simulink model "sysgenPolyphaseChannelizer"  (Simulink 7.7)
settings: Solver=VariableStepDiscrete  StartTime=0.0  StopTime=200000.0  RelTol=1e-3
values from neighbouring files (symbols this model uses):
  Fs = 1 ./ block_data.params.XIncr    [sdspfscope2_r13.m]
undefined symbols (not defined in the file or in its folder): sided, Two, xlfda_numerator, xlipgetpartsetting
libraries: xbsIndex_r4 x37, dspsigops x6, dspsrcs4 x3, dspsnks4 x2, simulink x1, xbsCopyrightNotice_r4 x1
settings Model: Creator=andrewd  LastModifiedBy=arvinds
settings OptimizationCC: InitFltsAndDblsToZero=on
settings DebuggingCC: SaveWithParameterizedLinksMsg=none  SignalResolutionControl=TryResolveAllWithWarning  StrictBusMsg=Warning
settings GRTTargetCC: TargetFcnLib=ansi_tfl_tmw.mat

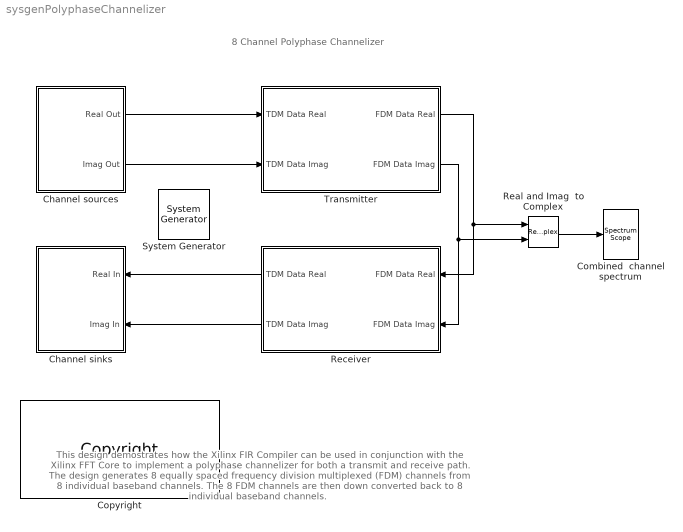
== system sysgenPolyphaseChannelizer ==
  note: 8 Channel Polyphase Channelizer
  note: This design demostrates how the Xilinx FIR Compiler can be used
      | in conjunction with the Xilinx FFT Core to implement a polyphase
      | channelizer for both a transmit and receive path.
      |
      | The design generates 8 equally spaced frequency division multiplexed
      | (FDM) channels from 8 individual baseband channels. The 8 FDM
      | channels are then down converted back to 8 individual baseband
      | channels.
  " System Generator" : xbsIndex_r4/ System Generator  Tag=genX  SystemSampleTime=-1  xilinxfamily=virtex6  part=xc6vlx240t  speed=-1  package=ff1156  synthesis_tool=XST  clock_wrapper=Clock Enables  directory=./timing  proj_type=Project Navigator  Synth_file=XST Defaults  Impl_file=ISE Defaults  testbench=off  simulink_period=1  sysclk_period=1e9/(length(xlfda_numerator([bdroot,'/Transmitter/FDATool']))*200e3)  dcm_input_clock_period=100  incr_netlist=off  trim_vbits=Everywhere in SubSystem  dbl_ovrd=According to Block Masks  core_generation=According to Block Masks  run_coregen=off  deprecated_control=off  eval_field=0  block_type=sysgen
      settings: block_version=10.1.2
  Channel sinks : Subsystem
  Channel sources : Subsystem
  Combined  channel spectrum : dspsnks4/Spectrum Scope  SystemSampleTime=-1  ScopeProperties=on  Domain=Frequency  HorizSpan=1  UseBuffer=on  BufferSize=512  Overlap=0  TreatMby1Signals=M channels  inpFftLenInherit=on  FFTlength=512  numAvg=2  DisplayProperties=off  AxisGrid=on  Memory=off  FrameNumber=on  AxisLegend=off  AxisZoom=off  OpenScopeAtSimStart=on  OpenScopeImmediately=off  FigPos=[-726 581 381 243]  AxisProperties=off  XUnits=Hertz  XRange=Two-sided ((-Fs/2...Fs/2])  XDisplay=0  InheritXIncr=on  XIncr=1.0  XLabel=Samples  XLimit=User-defined  YUnits=dBm/Hertz  XMax=0.005618  XMin=-0.005618  YLabel=Magnitude-squared, dB  LineProperties=off  wintypeSpecScope=Hann  RsSpecScope=50  betaSpecScope=5  winsampSpecScope=Periodic  XAxisParamsVer=6.8  isFrameUpgraded=on
      settings: YMin=-112.1379  YMax=9.2197
  Copyright : xbsCopyrightNotice_r4/Copyright  copyrighttext="Copyright (c) 2011  by  Xilinx, Inc. All rights reserved.<br><br>This file contains proprietary, confidential information of Xilinx, Inc., is distributed under license from Xilinx, Inc., and may be used, copied and/or disclosed only pursuant to the terms of a valid license agreement with Xilinx, Inc. Xilinx hereby grants you a license to use this file solely for design, simulation, implementation and creation of design files limited to Xilinx devices or technologies. Use with non-Xilinx devices or technologies is expressly prohibited and immediately terminates your license unless covered by a separate agreement.<br><br>Xilinx is providing this design, code, or information \"as-is\" solely for use in developing programs and solutions for Xilinx devices, with no obligation on the part of Xilinx to provide support. By providing this design, code, or information as one possible implementation of this feature, application or standard, Xilinx is making no representation that this implementation is free from any claims of infringement. You are responsible for obtaining any rights you may require for your implementation. Xilinx expressly disclaims any warranty whatsoever with respect to the adequacy of the implementation, including but not limited to any warranties or representations that this implementation is free from claims of infringement, implied warranties of merchantability or fitness for a particular purpose.<br><br>Xilinx products are not intended for use in life support appliances, devices, or systems. Use in such applications is expressly prohibited.<br><br>Any modifications that are made to the Source Code are done at the user's sole risk and will be unsupported.<br><br>This copyright and support notice must be retained as part of this text at all times. (c) Copyright 1995-2011 Xilinx, Inc. All rights reserved."  block_type=copyright
      settings: block_version=10.1.2
      settings: infoedit=|
      | Copyright(C) 2008 by  Xilinx, Inc. All rights reserved.<br>
      | <br>
      | This file contains proprietary, confidential information of Xilinx, Inc., is distributed under license
      | from Xilinx, Inc., and may be used, copied and/or disclosed only pursuant to the terms of a valid license
      | agreement with Xilinx, Inc. Xilinx hereby grants you a license to use this file solely for design,
      | simulation, implementation and creation of design files limited to Xilinx devices or technologies. Use
      | with non-Xilinx devices or technologies is expressly prohibited and immediately terminates your license
      | unless covered by a separate agreement.<br>
      | <br>
      | Xilinx is providing this design, code, or information "as-is" solely for use in developing programs and
      | solutions for Xilinx devices, with no obligation on the part of Xilinx to provide support. By providing
      | this design, code, or information as one possible implementation of this feature, application or standard,
      | Xilinx is making no representation that this implementation is free from any claims of infringement. You
      | are responsible for obtaining any rights you may require for your implementation. Xilinx expressly disclaims
      | any warranty whatsoever with respect to the adequacy of the implementation, including but not limited to any
      | warranties or representations that this implementation is free from claims of infringement, implied warranties
      | of merchantability or fitness for a particular purpose.<br>
      | <br>
      | Xilinx products are not intended for use in life support appliances, devices, or systems. Use in such
      | applications is expressly prohibited.<br>
      | <br>
      | Any modifications that are made to the Source Code are done at the user's sole risk and will be unsupported.<br>
      | <br>
      | This copyright and support notice must be retained as part of this text at all times.
      | (c) Copyright 1995-2008 Xilinx, Inc. All rights reserved.
  Real and Imag  to Complex : RealImagToComplex
  Receiver : Subsystem
  Transmitter : Subsystem
  wires:
  Channel sources/1(Real Out) -> Transmitter/1(TDM Data Real)
  Channel sources/2(Imag Out) -> Transmitter/2(TDM Data Imag)
  Real and Imag  to Complex/1 -> Combined  channel spectrum/1
  Transmitter/1(FDM Data Real) -> Receiver/1(FDM Data Real), Real and Imag  to Complex/1
  Transmitter/2(FDM Data Imag) -> Receiver/2(FDM Data Imag), Real and Imag  to Complex/2
  Receiver/1(TDM Data Real) -> Channel sinks/1(Real In)
  Receiver/2(TDM Data Imag) -> Channel sinks/2(Imag In)

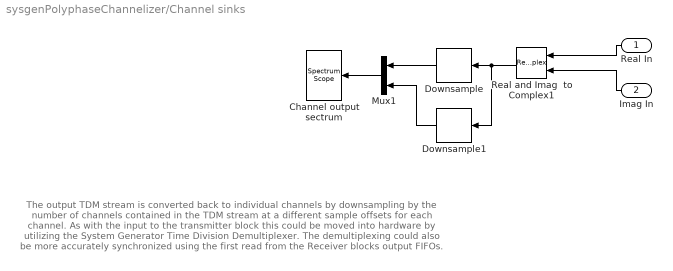
== system sysgenPolyphaseChannelizer/Channel sinks ==
  note: The output TDM stream is converted back to individual channels
      | by downsampling by the number of channels contained in the TDM
      | stream at a different sample offsets for each channel. As with the
      | input to the transmitter block this could be moved into hardware
      | by utilizing the System Generator Time Division Demultiplexer. The
      | demultiplexing could also be more accurately synchronized using
      | the first read from the Receiver blocks output FIFOs.
  Real In : Inport
  Imag In : Inport  Port=2
  Channel output sectrum : dspsnks4/Spectrum Scope  SystemSampleTime=-1  ScopeProperties=on  Domain=Frequency  HorizSpan=1  UseBuffer=on  BufferSize=256  Overlap=0  TreatMby1Signals=M channels  inpFftLenInherit=off  FFTlength=128  numAvg=2  DisplayProperties=off  AxisGrid=on  Memory=off  FrameNumber=on  AxisLegend=on  AxisZoom=off  OpenScopeAtSimStart=on  OpenScopeImmediately=off  FigPos=[-742 232 386 238]  AxisProperties=off  XUnits=Hertz  XRange=Two-sided ((-Fs/2...Fs/2])  XDisplay=0  InheritXIncr=on  XIncr=1.0  XLabel=Samples  XLimit=Auto  YUnits=dBm/Hertz  XMax=0.00070225  XMin=-0.00070225  YLabel=Magnitude-squared, dB  LineProperties=off  LineColors=[1 0 0]  wintypeSpecScope=Hann  RsSpecScope=50  betaSpecScope=5  winsampSpecScope=Periodic  XAxisParamsVer=6.9  isFrameUpgraded=on
      settings: YMin=-79.5628  YMax=47.0211
  Downsample : dspsigops/Downsample  N=8  phase=4  InputProcessing=Inherited (this choice will be removed - see release notes)  RateOptions=Enforce single-rate processing  smode=Allow multirate  fmode=Maintain input frame size  ic=0
  Downsample1 : dspsigops/Downsample  N=8  phase=0  InputProcessing=Inherited (this choice will be removed - see release notes)  RateOptions=Enforce single-rate processing  smode=Allow multirate  fmode=Maintain input frame size  ic=0
  Mux1 : Mux  Inputs=2
  Real and Imag  to Complex1 : RealImagToComplex
  wires:
  Real and Imag  to Complex1/1 -> Downsample/1, Downsample1/1
  Mux1/1 -> Channel output sectrum/1
  Downsample/1 -> Mux1/1
  Downsample1/1 -> Mux1/2
  Real In/1 -> Real and Imag  to Complex1/1
  Imag In/1 -> Real and Imag  to Complex1/2

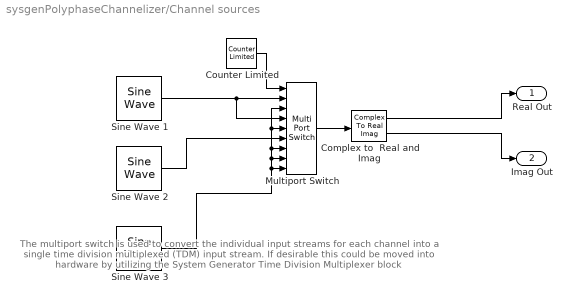
== system sysgenPolyphaseChannelizer/Channel sources ==
  note: The multiport switch is used to convert the individual input streams
      | for each channel into a single time division multiplexed (TDM)
      | input stream. If desirable this could be moved into hardware by
      | utilizing the System Generator Time Division Multiplexer block
  Complex to  Real and Imag : ComplexToRealImag
  Counter Limited : simulink/Sources/Counter Limited  SystemSampleTime=-1  uplimit=7  tsamp=length(xlfda_numerator([bdroot,'/Transmitter/FDATool']))/8
  Multiport Switch : MultiPortSwitch  DataPortOrder=Zero-based contiguous  Inputs=8  zeroidx=on  InputSameDT=on
  Sine Wave 1 : dspsrcs4/Sine Wave  Amplitude=1  Frequency=11.23456e3/(200e3*length(xlfda_numerator([bdroot,'/Transmitter/FDATool'])))  Phase=0  SampleMode=Discrete  OutComplex=Complex  CompMethod=Trigonometric fcn  TableSize=Speed  SampleTime=length(xlfda_numerator([bdroot,'/Transmitter/FDATool']))  SamplesPerFrame=1  ResetState=Restart at time zero  dataType=double  wordLen=16  udDataType=sfix(16)  fracBitsMode=Best precision  numFracBits=15  OutDataTypeStr=double  LastOutDataTypeStr=double
  Sine Wave 2 : dspsrcs4/Sine Wave  Amplitude=0.5  Frequency=50.234567e3/(200e3*length(xlfda_numerator([bdroot,'/Transmitter/FDATool'])))  Phase=0  SampleMode=Discrete  OutComplex=Complex  CompMethod=Trigonometric fcn  TableSize=Speed  SampleTime=length(xlfda_numerator([bdroot,'/Transmitter/FDATool']))  SamplesPerFrame=1  ResetState=Restart at time zero  dataType=double  wordLen=16  udDataType=sfix(16)  fracBitsMode=Best precision  numFracBits=15  OutDataTypeStr=double  LastOutDataTypeStr=double
  Sine Wave 3 : dspsrcs4/Sine Wave  Amplitude=0  Frequency=0  Phase=0  SampleMode=Discrete  OutComplex=Complex  CompMethod=Trigonometric fcn  TableSize=Speed  SampleTime=length(xlfda_numerator([bdroot,'/Transmitter/FDATool']))  SamplesPerFrame=1  ResetState=Restart at time zero  dataType=double  wordLen=16  udDataType=sfix(16)  fracBitsMode=Best precision  numFracBits=15  OutDataTypeStr=double  LastOutDataTypeStr=double
  Real Out : Outport
  Imag Out : Outport  Port=2
  wires:
  Multiport Switch/1 -> Complex to  Real and Imag/1
  Sine Wave 1/1 -> Multiport Switch/2, Multiport Switch/4
  Counter Limited/1 -> Multiport Switch/1
  Sine Wave 2/1 -> Multiport Switch/6
  Sine Wave 3/1 -> Multiport Switch/8, Multiport Switch/7, Multiport Switch/5, Multiport Switch/3, Multiport Switch/9
  Complex to  Real and Imag/1 -> Real Out/1
  Complex to  Real and Imag/2 -> Imag Out/1

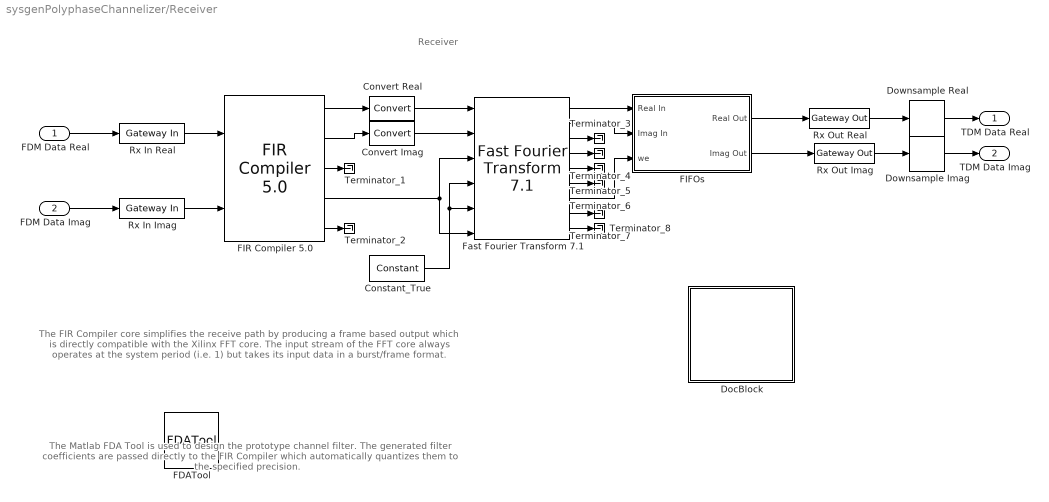
== system sysgenPolyphaseChannelizer/Receiver ==
  note: The FIR Compiler core simplifies the receive path by producing a frame
      | based output which is directly compatible with the Xilinx FFT core.
      | The input stream of the FFT core always operates at the system
      | period (i.e. 1) but takes its input data in a burst/frame format.
  note: Receiver
  note: The Matlab FDA Tool is used to design the prototype
      | channel filter. The generated filter coefficients are
      | passed directly to the FIR Compiler which
      | automatically quantizes them to the specified
      | precision.
  FDM Data Real : Inport
  FDM Data Imag : Inport  Port=2
  Constant_True : xbsIndex_r4/Constant  const=1  gui_display_data_type=Fixed-point  arith_type=Boolean  n_bits=16  bin_pt=14  preci_type=Single  exp_width=8  frac_width=24  explicit_period=on  period=1  equ=P=C  opselect=C  inp2=PCIN>>17  opr=+  inp1=P  carry=CIN  dbl_ovrd=off  block_type=constant
      settings: block_version=10.1.2
  Convert Imag : xbsIndex_r4/Convert  gui_display_data_type=Fixed-point  arith_type="Signed  (2's comp)"  n_bits=17  bin_pt=16  float_type=Single  exp_bits=8  fraction_bits=24  quantization=Truncate  overflow=Wrap  en=off  latency=0  dbl_ovrd=off  pipeline=off  block_type=convert
      settings: block_version=10.1.2
  Convert Real : xbsIndex_r4/Convert  gui_display_data_type=Fixed-point  arith_type="Signed  (2's comp)"  n_bits=17  bin_pt=16  float_type=Single  exp_bits=8  fraction_bits=24  quantization=Truncate  overflow=Wrap  en=off  latency=0  dbl_ovrd=off  pipeline=off  block_type=convert
      settings: block_version=10.1.2
  DocBlock : Subsystem  AncestorBlock=simulink/Model-Wide Utilities/DocBlock  mask(DocBlock){ECoderFlag=, DocumentType=RTF}
      mask prompts: ECoderFlag "RTW Embedded Coder Flag"; DocumentType "Document Type"
      mask help: Use this block to save long descriptive text with the model. Double-clicking the block will open an editor.
      settings: DeleteFcn=docblock('close_document',gcb);  PreSaveFcn=docblock('save_document',gcb);  OpenFcn=docblock('edit_document',gcb);
      mask StyleString: edit,popup(Text|RTF|HTML)
      mask Display:
      | plot([.8 0 0 1 1 .8 .8 1],[1 1 0 0 .8 1 .8 .8]);
      | text(.5,.6,'Double click\n for more information','horizontalalignment','center');
  Downsample Imag : dspsigops/Downsample  N=length(xlfda_numerator('FDATool'))/8  phase=0  InputProcessing=Inherited (this choice will be removed - see release notes)  RateOptions=Enforce single-rate processing  smode=Allow multirate  fmode=Maintain input frame size  ic=0
  Downsample Real : dspsigops/Downsample  N=length(xlfda_numerator('FDATool'))/8  phase=0  InputProcessing=Inherited (this choice will be removed - see release notes)  RateOptions=Enforce single-rate processing  smode=Allow multirate  fmode=Maintain input frame size  ic=0
  FDATool : xbsIndex_r4/FDATool  block_type=fdatool
      settings: infoedit=FDATool  block_version=10.1.2
  FIFOs : Subsystem
  "FIR Compiler 5.0 " : xbsIndex_r4/FIR Compiler 5.0   coefficientvector=8.*xlfda_numerator('FDATool')  coefficient_sets=1  filter_type=Polyphase_Filter_Bank_Receiver  rate_change_type=Integer  interpolation_rate=1  decimation_rate=1  zero_pack_factor=1  number_channels=8  ratespecification=Maximum_Possible  sampleperiod=1  hardwareoversamplingrate=1  filter_architecture=Systolic_Multiply_Accumulate  coefficient_reload=off  coefficient_structure=Non_Symmetric  coefficient_sign=Signed  quantization=Quantize_Only  coefficient_width=25  bestprecision=off  coefficient_fractional_bits=24  number_paths=2  output_rounding_mode=Convergent_Rounding_to_Even  output_width=19  allow_rounding_approximation=off  optimization_goal=Area  has_sclr=off  has_data_valid=off  has_nd=off  has_ce=off  usechan_in_adv=off  chan_in_adv=0  data_buffer_type=Automatic  coefficient_buffer_type=Automatic  input_buffer_type=Automatic  output_buffer_type=Automatic  preference_for_other_storage=Automatic  multi_column_support=Automatic  columnconfig='32,32,25'  inter_column_pipe_length=4  passband_min=0.0  passband_max=0.5  stopband_min=0.5  stopband_max=1.0  filter_selection=1  gui_behaviour=Sysgen  registered_output=true  data_sign=Signed  data_width=16  data_fractional_bits=0  wrapper_available=true  ip_wrap_arbitrary_binary_point=true  ip_name=FIR Compiler  ip_version=5.0  dsptool_ready=true  ipcore_usecache=true  ipcore_useipmodelcache=true  ipcore_xco_need_fpga_part=true  port_translation_map={ 'ce' => 'en', 'sclr' => 'rst' }  run_core_at_system_period=true  ipcore_fpga_part=xlipgetpartsetting(gcb, {'virtex4', 'xc4vsx35', '-10', 'ff668'})  structural_sim=false  block_type=fir_compiler_v5_0
      settings: block_version=11.1.2
  "Fast Fourier Transform 7.1 " : xbsIndex_r4/Fast Fourier Transform 7.1   transform_length=8  implementation_options=radix_2_lite_burst_io  target_clock_frequency=250  target_data_throughput=50  run_time_configurable_transform_length=off  phase_factor_width=17  scaling_options=unscaled  rounding_modes=convergent_rounding  output_ordering=natural_order  cyclic_prefix_insertion=off  ce=off  sclr=off  ovflo=off  input_data_offset=three_cycle_offset  memory_options_data=distributed_ram  memory_options_phase_factors=distributed_ram  number_of_stages_using_block_ram_for_data_and_phase_factors=0  memory_options_reorder=block_ram  memory_options_hybrid=off  complex_mult_type=use_mults_performance  butterfly_type=use_xtremedsp_slices  channels=1  input_ordering=natural_order  input_width=16  simulation_type=external_xfix  simulation_model=fftv71_CModel:fftv71_cmodel  ip_name=Fast Fourier Transform  ip_version=7.1  dsptool_ready=true  wrapper_available=true  port_translation_map={ 'ce' => 'en', 'sclr' => 'rst' }  ipcore_fpga_part=xlipgetpartsetting(gcb, {'virtex4', 'xc4vsx35', '-10', 'ff668'})  block_type=xfft_v7_1
      settings: block_version=12.1
  Rx In Imag : xbsIndex_r4/Gateway In  gui_display_data_type=Fixed-point  arith_type="Signed  (2's comp)"  n_bits=16  bin_pt=15  preci_type=Single  exp_width=8  frac_width=24  quantization="Round  (unbiased: +/- Inf)"  overflow=Saturate  period=length(xlfda_numerator('FDATool'))/8  dbl_ovrd=off  timing_constraint=None  locs_specified=off  LOCs={}  inherit_from_input=off  UseAsADC=off  ADCChannel='1'  hdl_port=on  block_type=gatewayin
      settings: infoedit="Gateway in block.  Converts inputs of type Simulink integer, double and fixed point to  Xilinx fixed point type.<P><P>Hardware notes:  In hardware these blocks become top level input ports."  block_version=10.1.2
  Rx In Real : xbsIndex_r4/Gateway In  gui_display_data_type=Fixed-point  arith_type="Signed  (2's comp)"  n_bits=16  bin_pt=15  preci_type=Single  exp_width=8  frac_width=24  quantization="Round  (unbiased: +/- Inf)"  overflow=Saturate  period=length(xlfda_numerator('FDATool'))/8  dbl_ovrd=off  timing_constraint=None  locs_specified=off  LOCs={}  inherit_from_input=off  UseAsADC=off  ADCChannel='1'  hdl_port=on  block_type=gatewayin
      settings: infoedit="Gateway in block.  Converts inputs of type Simulink integer, double and fixed point to  Xilinx fixed point type.<P><P>Hardware notes:  In hardware these blocks become top level input ports."  block_version=10.1.2
  Rx Out Imag : xbsIndex_r4/Gateway Out  inherit_from_input=off  hdl_port=on  timing_constraint=None  locs_specified=off  LOCs={}  UseAsDAC=off  DACChannel='1'  block_type=gatewayout
      settings: infoedit="Gateway out block.  Converts Xilinx fixed point inputs into ouputs of type Simulink integer, double, or fixed point.<P><P>Hardware notes:  In hardware these blocks become top level output ports or are discarded, depending on how they are configured."  block_version=10.1.2
  Rx Out Real : xbsIndex_r4/Gateway Out  inherit_from_input=off  hdl_port=on  timing_constraint=None  locs_specified=off  LOCs={}  UseAsDAC=off  DACChannel='1'  block_type=gatewayout
      settings: infoedit="Gateway out block.  Converts Xilinx fixed point inputs into ouputs of type Simulink integer, double, or fixed point.<P><P>Hardware notes:  In hardware these blocks become top level output ports or are discarded, depending on how they are configured."  block_version=10.1.2
  Terminator_{1..8} (8 alike) : Terminator
  TDM Data Real : Outport
  TDM Data Imag : Outport  Port=2
  wires:
  FDM Data Real/1 -> Rx In Real/1
  FDM Data Imag/1 -> Rx In Imag/1
  Rx In Real/1 -> "FIR Compiler 5.0 "/1
  Rx In Imag/1 -> "FIR Compiler 5.0 "/2
  "FIR Compiler 5.0 "/1 -> Convert Real/1
  "FIR Compiler 5.0 "/2 -> Convert Imag/1
  Constant_True/1 -> "Fast Fourier Transform 7.1 "/5, "Fast Fourier Transform 7.1 "/4
  Convert Real/1 -> "Fast Fourier Transform 7.1 "/1
  Convert Imag/1 -> "Fast Fourier Transform 7.1 "/2
  "FIR Compiler 5.0 "/4 -> "Fast Fourier Transform 7.1 "/6, "Fast Fourier Transform 7.1 "/3
  "Fast Fourier Transform 7.1 "/1 -> FIFOs/1(Real In)
  "Fast Fourier Transform 7.1 "/2 -> FIFOs/2(Imag In)
  "Fast Fourier Transform 7.1 "/7 -> FIFOs/3(we)
  FIFOs/1(Real Out) -> Rx Out Real/1
  FIFOs/2(Imag Out) -> Rx Out Imag/1
  Rx Out Real/1 -> Downsample Real/1
  Rx Out Imag/1 -> Downsample Imag/1
  "FIR Compiler 5.0 "/3 -> Terminator_1/1
  "FIR Compiler 5.0 "/5 -> Terminator_2/1
  "Fast Fourier Transform 7.1 "/3 -> Terminator_3/1
  "Fast Fourier Transform 7.1 "/4 -> Terminator_4/1
  "Fast Fourier Transform 7.1 "/5 -> Terminator_5/1
  "Fast Fourier Transform 7.1 "/6 -> Terminator_6/1
  "Fast Fourier Transform 7.1 "/8 -> Terminator_7/1
  "Fast Fourier Transform 7.1 "/9 -> Terminator_8/1
  Downsample Real/1 -> TDM Data Real/1
  Downsample Imag/1 -> TDM Data Imag/1

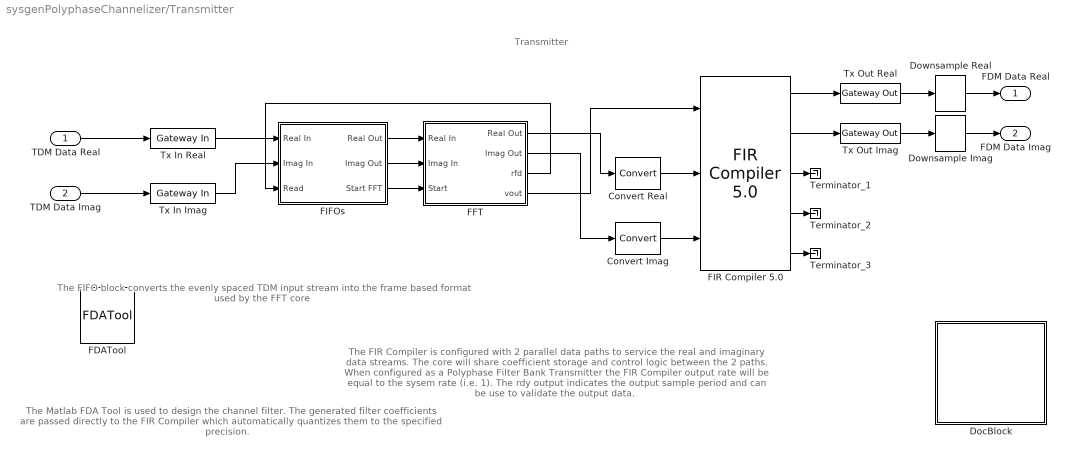
== system sysgenPolyphaseChannelizer/Transmitter ==
  note: The FIFO block converts the evenly spaced
      | TDM input stream into the frame based format
      | used by the FFT core
  note: The FIR Compiler is configured with 2 parallel data paths
      | to service the real and imaginary data streams. The core will
      | share coefficient storage and control logic between the 2 paths.
      | When configured as a Polyphase Filter Bank Transmitter the
      | FIR Compiler output rate will be equal to the sysem rate (i.e. 1).
      | The rdy output indicates the output sample period and can be
      | use to validate the output data.
  note: Transmitter
  note: The Matlab FDA Tool is used to design the
      | channel filter. The generated filter coefficients are
      | passed directly to the FIR Compiler which
      | automatically quantizes them to the specified
      | precision.
  TDM Data Real : Inport
  TDM Data Imag : Inport  Port=2
  Convert Imag : xbsIndex_r4/Convert  gui_display_data_type=Fixed-point  arith_type="Signed  (2's comp)"  n_bits=18  bin_pt=13  float_type=Single  exp_bits=8  fraction_bits=24  quantization="Round  (unbiased: Even Values)"  overflow=Wrap  en=off  latency=0  dbl_ovrd=off  pipeline=off  block_type=convert
      settings: block_version=10.1.2
  Convert Real : xbsIndex_r4/Convert  gui_display_data_type=Fixed-point  arith_type="Signed  (2's comp)"  n_bits=18  bin_pt=13  float_type=Single  exp_bits=8  fraction_bits=24  quantization="Round  (unbiased: Even Values)"  overflow=Wrap  en=off  latency=0  dbl_ovrd=off  pipeline=off  block_type=convert
      settings: block_version=10.1.2
  DocBlock : Subsystem  AncestorBlock=simulink/Model-Wide Utilities/DocBlock  mask(DocBlock){ECoderFlag=, DocumentType=RTF}
      mask prompts: ECoderFlag "RTW Embedded Coder Flag"; DocumentType "Document Type"
      mask help: Use this block to save long descriptive text with the model. Double-clicking the block will open an editor.
      settings: DeleteFcn=docblock('close_document',gcb);  PreSaveFcn=docblock('save_document',gcb);  OpenFcn=docblock('edit_document',gcb);
      mask StyleString: edit,popup(Text|RTF|HTML)
      mask Display:
      | plot([.8 0 0 1 1 .8 .8 1],[1 1 0 0 .8 1 .8 .8]);
      | text(.5,.6,'Double click\n for more information','horizontalalignment','center');
  Downsample Imag : dspsigops/Downsample  N=length(xlfda_numerator('FDATool'))/8  phase=0  InputProcessing=Inherited (this choice will be removed - see release notes)  RateOptions=Enforce single-rate processing  smode=Allow multirate  fmode=Maintain input frame size  ic=0
  Downsample Real : dspsigops/Downsample  N=length(xlfda_numerator('FDATool'))/8  phase=0  InputProcessing=Inherited (this choice will be removed - see release notes)  RateOptions=Enforce single-rate processing  smode=Allow multirate  fmode=Maintain input frame size  ic=0
  FDATool : xbsIndex_r4/FDATool  block_type=fdatool
      settings: infoedit=FDATool  block_version=10.1.2
  FFT : Subsystem
  FIFOs : Subsystem
  "FIR Compiler 5.0 " : xbsIndex_r4/FIR Compiler 5.0   coefficientvector=xlfda_numerator('FDATool')  coefficient_sets=1  filter_type=Polyphase_Filter_Bank_Transmitter  rate_change_type=Integer  interpolation_rate=1  decimation_rate=1  zero_pack_factor=1  number_channels=8  ratespecification=Sample_Period  sampleperiod=length(xlfda_numerator('FDATool'))/8  hardwareoversamplingrate=1  filter_architecture=Systolic_Multiply_Accumulate  coefficient_reload=off  coefficient_structure=Non_Symmetric  coefficient_sign=Signed  quantization=Quantize_Only  coefficient_width=25  bestprecision=off  coefficient_fractional_bits=27  number_paths=2  output_rounding_mode=Convergent_Rounding_to_Odd  output_width=19  allow_rounding_approximation=off  optimization_goal=Area  has_sclr=off  has_data_valid=off  has_nd=on  has_ce=off  usechan_in_adv=off  chan_in_adv=0  data_buffer_type=Automatic  coefficient_buffer_type=Automatic  input_buffer_type=Automatic  output_buffer_type=Automatic  preference_for_other_storage=Automatic  multi_column_support=Disabled  columnconfig='1'  inter_column_pipe_length=4  passband_min=0.0  passband_max=0.5  stopband_min=0.5  stopband_max=1.0  filter_selection=1  gui_behaviour=Sysgen  registered_output=true  data_sign=Signed  data_width=16  data_fractional_bits=0  wrapper_available=true  ip_wrap_arbitrary_binary_point=true  ip_name=FIR Compiler  ip_version=5.0  dsptool_ready=true  ipcore_usecache=true  ipcore_useipmodelcache=true  ipcore_xco_need_fpga_part=true  port_translation_map={ 'ce' => 'en', 'sclr' => 'rst' }  run_core_at_system_period=true  ipcore_fpga_part=xlipgetpartsetting(gcb, {'virtex4', 'xc4vsx35', '-10', 'ff668'})  structural_sim=false  block_type=fir_compiler_v5_0
      settings: block_version=11.1.2
  Terminator_1 : Terminator
  Terminator_2 : Terminator
  Terminator_3 : Terminator
  Tx In Imag : xbsIndex_r4/Gateway In  gui_display_data_type=Fixed-point  arith_type="Signed  (2's comp)"  n_bits=15  bin_pt=14  preci_type=Single  exp_width=8  frac_width=24  quantization="Round  (unbiased: +/- Inf)"  overflow=Saturate  period=length(xlfda_numerator('FDATool'))/8  dbl_ovrd=off  timing_constraint=None  locs_specified=off  LOCs={}  inherit_from_input=off  UseAsADC=off  ADCChannel='1'  hdl_port=on  block_type=gatewayin
      settings: infoedit="Gateway in block.  Converts inputs of type Simulink integer, double and fixed point to  Xilinx fixed point type.<P><P>Hardware notes:  In hardware these blocks become top level input ports."  block_version=10.1.2
  Tx In Real : xbsIndex_r4/Gateway In  gui_display_data_type=Fixed-point  arith_type="Signed  (2's comp)"  n_bits=15  bin_pt=14  preci_type=Single  exp_width=8  frac_width=24  quantization="Round  (unbiased: +/- Inf)"  overflow=Saturate  period=length(xlfda_numerator('FDATool'))/8  dbl_ovrd=off  timing_constraint=None  locs_specified=off  LOCs={}  inherit_from_input=off  UseAsADC=off  ADCChannel='1'  hdl_port=on  block_type=gatewayin
      settings: infoedit="Gateway in block.  Converts inputs of type Simulink integer, double and fixed point to  Xilinx fixed point type.<P><P>Hardware notes:  In hardware these blocks become top level input ports."  block_version=10.1.2
  Tx Out Imag : xbsIndex_r4/Gateway Out  inherit_from_input=off  hdl_port=on  timing_constraint=None  locs_specified=off  LOCs={}  UseAsDAC=off  DACChannel='1'  block_type=gatewayout
      settings: infoedit="Gateway out block.  Converts Xilinx fixed point inputs into ouputs of type Simulink integer, double, or fixed point.<P><P>Hardware notes:  In hardware these blocks become top level output ports or are discarded, depending on how they are configured."  block_version=10.1.2
  Tx Out Real : xbsIndex_r4/Gateway Out  inherit_from_input=off  hdl_port=on  timing_constraint=None  locs_specified=off  LOCs={}  UseAsDAC=off  DACChannel='1'  block_type=gatewayout
      settings: infoedit="Gateway out block.  Converts Xilinx fixed point inputs into ouputs of type Simulink integer, double, or fixed point.<P><P>Hardware notes:  In hardware these blocks become top level output ports or are discarded, depending on how they are configured."  block_version=10.1.2
  FDM Data Real : Outport
  FDM Data Imag : Outport  Port=2
  wires:
  TDM Data Real/1 -> Tx In Real/1
  TDM Data Imag/1 -> Tx In Imag/1
  Tx In Real/1 -> FIFOs/1(Real In)
  Tx In Imag/1 -> FIFOs/2(Imag In)
  FIFOs/1(Real Out) -> FFT/1(Real In)
  FIFOs/2(Imag Out) -> FFT/2(Imag In)
  FIFOs/3(Start FFT) -> FFT/3(Start)
  FFT/3(rfd) -> FIFOs/3(Read)
  Convert Real/1 -> "FIR Compiler 5.0 "/2
  Convert Imag/1 -> "FIR Compiler 5.0 "/3
  FFT/1(Real Out) -> Convert Real/1
  FFT/2(Imag Out) -> Convert Imag/1
  Tx Out Real/1 -> Downsample Real/1
  Tx Out Imag/1 -> Downsample Imag/1
  "FIR Compiler 5.0 "/1 -> Tx Out Real/1
  "FIR Compiler 5.0 "/2 -> Tx Out Imag/1
  FFT/4(vout) -> "FIR Compiler 5.0 "/1
  Downsample Real/1 -> FDM Data Real/1
  Downsample Imag/1 -> FDM Data Imag/1
  "FIR Compiler 5.0 "/3 -> Terminator_1/1
  "FIR Compiler 5.0 "/4 -> Terminator_2/1
  "FIR Compiler 5.0 "/5 -> Terminator_3/1

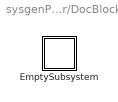
== system sysgenPolyphaseChannelizer/Receiver/DocBlock ==
  EmptySubsystem : Subsystem

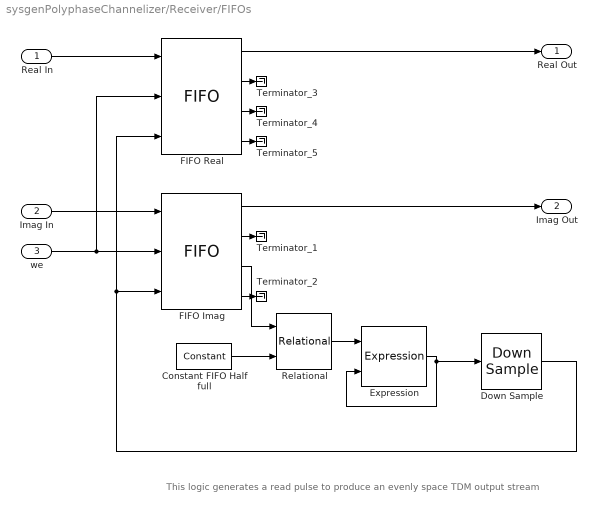
== system sysgenPolyphaseChannelizer/Receiver/FIFOs ==
  note: This logic generates a read pulse to produce an evenly space TDM output stream
  Real In : Inport
  Imag In : Inport  Port=2
  we : Inport  Port=3
  Constant FIFO Half full : xbsIndex_r4/Constant  const=0.5  gui_display_data_type=Fixed-point  arith_type=Unsigned  n_bits=1  bin_pt=1  preci_type=Single  exp_width=8  frac_width=24  explicit_period=on  period=length(xlfda_numerator('../FDATool'))/8  equ=P=C  opselect=C  inp2=PCIN>>17  opr=+  inp1=P  carry=CIN  dbl_ovrd=off  block_type=constant
      settings: block_version=10.1.2
  Down Sample : xbsIndex_r4/Down Sample  sample_ratio=length(xlfda_numerator('../FDATool'))/8  sample_phase=First Value of Frame  en=off  latency=0  dbl_ovrd=off  block_type=dsamp
      settings: block_version=10.1.2
  Expression : xbsIndex_r4/Expression  expression=a|b  align_bp=on  en=off  latency=1  precision=Full  arith_type=Unsigned  n_bits=16  bin_pt=0  dbl_ovrd=off  block_type=expr
      settings: block_version=10.1.2
  FIFO Imag : xbsIndex_r4/FIFO  performance_options=Standard_FIFO  depth=16  percent_nbits=1  rst=off  en=off  use_dcount=off  use_percent_full_port=on  use_almost_empty=off  almost_empty_thresh=2  use_almost_full=off  almost_full_thresh=8  dbl_ovrd=off  mem_type=Block RAM  explicit_period=off  block_type=fifo
      settings: block_version=10.1.2
  FIFO Real : xbsIndex_r4/FIFO  performance_options=Standard_FIFO  depth=16  percent_nbits=1  rst=off  en=off  use_dcount=off  use_percent_full_port=on  use_almost_empty=off  almost_empty_thresh=2  use_almost_full=off  almost_full_thresh=8  dbl_ovrd=off  mem_type=Block RAM  explicit_period=off  block_type=fifo
      settings: block_version=10.1.2
  Relational : xbsIndex_r4/Relational  mode=a=b  en=off  latency=0  dbl_ovrd=off  block_type=relational
      settings: block_version=10.1.2
  Terminator_{1..5} (5 alike) : Terminator
  Real Out : Outport
  Imag Out : Outport  Port=2
  wires:
  Relational/1 -> Expression/1
  Constant FIFO Half full/1 -> Relational/2
  Real In/1 -> FIFO Real/1
  Imag In/1 -> FIFO Imag/1
  we/1 -> FIFO Imag/2, FIFO Real/2
  FIFO Imag/3 -> Relational/1
  Expression/1 -> Expression/2, Down Sample/1
  Down Sample/1 -> FIFO Real/3, FIFO Imag/3
  FIFO Real/1 -> Real Out/1
  FIFO Imag/1 -> Imag Out/1
  FIFO Imag/2 -> Terminator_1/1
  FIFO Imag/4 -> Terminator_2/1
  FIFO Real/2 -> Terminator_3/1
  FIFO Real/3 -> Terminator_4/1
  FIFO Real/4 -> Terminator_5/1

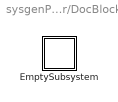
== system sysgenPolyphaseChannelizer/Transmitter/DocBlock ==
  EmptySubsystem : Subsystem

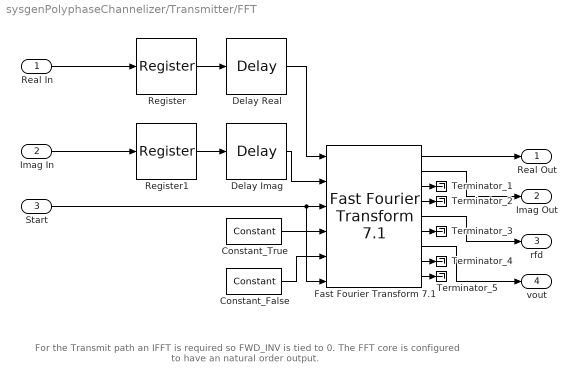
== system sysgenPolyphaseChannelizer/Transmitter/FFT ==
  note: For the Transmit path an IFFT is required so FWD_INV is tied
      | to 0. The FFT core is configured to have an natural order output.
  Real In : Inport
  Imag In : Inport  Port=2
  Start : Inport  Port=3
  Constant_False : xbsIndex_r4/Constant  const=0  gui_display_data_type=Fixed-point  arith_type=Boolean  n_bits=16  bin_pt=14  preci_type=Single  exp_width=8  frac_width=24  explicit_period=on  period=1  equ=P=C  opselect=C  inp2=PCIN>>17  opr=+  inp1=P  carry=CIN  dbl_ovrd=off  block_type=constant
      settings: block_version=10.1.2
  Constant_True : xbsIndex_r4/Constant  const=1  gui_display_data_type=Fixed-point  arith_type=Boolean  n_bits=16  bin_pt=14  preci_type=Single  exp_width=8  frac_width=24  explicit_period=on  period=1  equ=P=C  opselect=C  inp2=PCIN>>17  opr=+  inp1=P  carry=CIN  dbl_ovrd=off  block_type=constant
      settings: block_version=10.1.2
  Delay Imag : xbsIndex_r4/Delay  rst=off  infoeditControl=Selection of Reset will increase slice count due to use of real FFs and instead of SRLs  en=off  latency=1  dbl_ovrd=off  reg_retiming=off  block_type=delay
      settings: block_version=10.1.2
  Delay Real : xbsIndex_r4/Delay  rst=off  infoeditControl=Selection of Reset will increase slice count due to use of real FFs and instead of SRLs  en=off  latency=1  dbl_ovrd=off  reg_retiming=off  block_type=delay
      settings: block_version=10.1.2
  "Fast Fourier Transform 7.1 " : xbsIndex_r4/Fast Fourier Transform 7.1   transform_length=8  implementation_options=radix_2_lite_burst_io  target_clock_frequency=250  target_data_throughput=50  run_time_configurable_transform_length=off  phase_factor_width=17  scaling_options=unscaled  rounding_modes=convergent_rounding  output_ordering=natural_order  cyclic_prefix_insertion=off  ce=off  sclr=off  ovflo=off  input_data_offset=three_cycle_offset  memory_options_data=distributed_ram  memory_options_phase_factors=distributed_ram  number_of_stages_using_block_ram_for_data_and_phase_factors=0  memory_options_reorder=block_ram  memory_options_hybrid=off  complex_mult_type=use_mults_performance  butterfly_type=use_xtremedsp_slices  channels=1  input_ordering=natural_order  input_width=16  simulation_type=external_xfix  simulation_model=fftv71_CModel:fftv71_cmodel  ip_name=Fast Fourier Transform  ip_version=7.1  dsptool_ready=true  wrapper_available=true  port_translation_map={ 'ce' => 'en', 'sclr' => 'rst' }  ipcore_fpga_part=xlipgetpartsetting(gcb, {'virtex4', 'xc4vsx35', '-10', 'ff668'})  block_type=xfft_v7_1
      settings: block_version=12.1
  Register : xbsIndex_r4/Register  init=0  rst=off  en=off  dbl_ovrd=off  block_type=register
      settings: block_version=11.1.2
  Register1 : xbsIndex_r4/Register  init=0  rst=off  en=off  dbl_ovrd=off  block_type=register
      settings: block_version=11.1.2
  Terminator_{1..5} (5 alike) : Terminator
  Real Out : Outport
  Imag Out : Outport  Port=2
  rfd : Outport  Port=3
  vout : Outport  Port=4
  wires:
  Delay Real/1 -> "Fast Fourier Transform 7.1 "/1
  Delay Imag/1 -> "Fast Fourier Transform 7.1 "/2
  Constant_True/1 -> "Fast Fourier Transform 7.1 "/4
  Real In/1 -> Register/1
  Imag In/1 -> Register1/1
  Start/1 -> "Fast Fourier Transform 7.1 "/3, "Fast Fourier Transform 7.1 "/6
  "Fast Fourier Transform 7.1 "/1 -> Real Out/1
  "Fast Fourier Transform 7.1 "/2 -> Imag Out/1
  "Fast Fourier Transform 7.1 "/5 -> rfd/1
  "Fast Fourier Transform 7.1 "/7 -> vout/1
  Constant_False/1 -> "Fast Fourier Transform 7.1 "/5
  "Fast Fourier Transform 7.1 "/3 -> Terminator_1/1
  "Fast Fourier Transform 7.1 "/4 -> Terminator_2/1
  "Fast Fourier Transform 7.1 "/6 -> Terminator_3/1
  "Fast Fourier Transform 7.1 "/8 -> Terminator_4/1
  "Fast Fourier Transform 7.1 "/9 -> Terminator_5/1
  Register/1 -> Delay Real/1
  Register1/1 -> Delay Imag/1

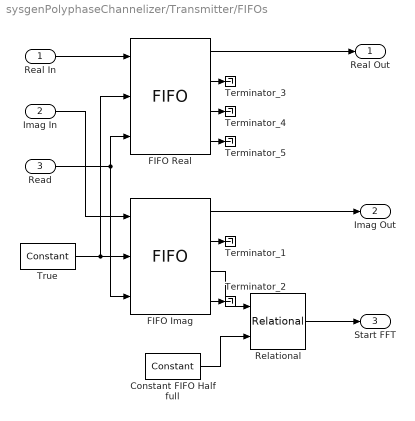
== system sysgenPolyphaseChannelizer/Transmitter/FIFOs ==
  Real In : Inport
  Imag In : Inport  Port=2
  Read : Inport  Port=3
  Constant FIFO Half full : xbsIndex_r4/Constant  const=0.5  gui_display_data_type=Fixed-point  arith_type=Unsigned  n_bits=1  bin_pt=1  preci_type=Single  exp_width=8  frac_width=24  explicit_period=on  period=1  equ=P=C  opselect=C  inp2=PCIN>>17  opr=+  inp1=P  carry=CIN  dbl_ovrd=off  block_type=constant
      settings: block_version=10.1.2
  FIFO Imag : xbsIndex_r4/FIFO  performance_options=Standard_FIFO  depth=16  percent_nbits=1  rst=off  en=off  use_dcount=off  use_percent_full_port=on  use_almost_empty=off  almost_empty_thresh=2  use_almost_full=off  almost_full_thresh=8  dbl_ovrd=off  mem_type=Block RAM  explicit_period=off  block_type=fifo
      settings: block_version=10.1.2
  FIFO Real : xbsIndex_r4/FIFO  performance_options=Standard_FIFO  depth=16  percent_nbits=1  rst=off  en=off  use_dcount=off  use_percent_full_port=on  use_almost_empty=off  almost_empty_thresh=2  use_almost_full=off  almost_full_thresh=8  dbl_ovrd=off  mem_type=Block RAM  explicit_period=off  block_type=fifo
      settings: block_version=10.1.2
  Relational : xbsIndex_r4/Relational  mode=a=b  en=off  latency=0  dbl_ovrd=off  block_type=relational
      settings: block_version=10.1.2
  Terminator_{1..5} (5 alike) : Terminator
  True : xbsIndex_r4/Constant  const=1  gui_display_data_type=Fixed-point  arith_type=Boolean  n_bits=16  bin_pt=14  preci_type=Single  exp_width=8  frac_width=24  explicit_period=on  period=length(xlfda_numerator('../FDATool'))/8  equ=P=C  opselect=C  inp2=PCIN>>17  opr=+  inp1=P  carry=CIN  dbl_ovrd=off  block_type=constant
      settings: block_version=10.1.2
  Real Out : Outport
  Imag Out : Outport  Port=2
  Start FFT : Outport  Port=3
  wires:
  Real In/1 -> FIFO Real/1
  Imag In/1 -> FIFO Imag/1
  Read/1 -> FIFO Real/3, FIFO Imag/3
  True/1 -> FIFO Imag/2, FIFO Real/2
  FIFO Imag/3 -> Relational/1
  Constant FIFO Half full/1 -> Relational/2
  Relational/1 -> Start FFT/1
  FIFO Real/1 -> Real Out/1
  FIFO Imag/1 -> Imag Out/1
  FIFO Imag/2 -> Terminator_1/1
  FIFO Imag/4 -> Terminator_2/1
  FIFO Real/2 -> Terminator_3/1
  FIFO Real/3 -> Terminator_4/1
  FIFO Real/4 -> Terminator_5/1

== system sysgenPolyphaseChannelizer/Receiver/DocBlock/EmptySubsystem ==

== system sysgenPolyphaseChannelizer/Transmitter/DocBlock/EmptySubsystem ==
